simulink model "left_arm_observer"  (R2019b)
settings: Solver=ode4  StartTime=0.0  StopTime=inf  FixedStep=0.001  MaxStep=0.01  RelTol=1e-3
model workspace (MAT data in the model file):
  SL_ROS_VariableLengthArrays_MaxSizes.CommonInfo.ArrayTruncateAction = 'EmitWarning'
  SL_ROS_VariableLengthArrays_MaxSizes.MsgTypeMap = containers.Map
  SL_ROS_VariableLengthArrays_MaxSizes.MsgTypeMap.serialization.keys = {'sensor_msgs/JointState', 'std_msgs/Float64MultiArray', 'std_msgs/String'}
  SL_ROS_VariableLengthArrays_MaxSizes.MsgTypeMap.serialization.values{1}(1).PropertyName = 'Effort'
  SL_ROS_VariableLengthArrays_MaxSizes.MsgTypeMap.serialization.values{1}(1).DataType = 'double'
  SL_ROS_VariableLengthArrays_MaxSizes.MsgTypeMap.serialization.values{1}(1).MaxLength = 7
  SL_ROS_VariableLengthArrays_MaxSizes.MsgTypeMap.serialization.values{1}(2).PropertyName = 'Name'
  SL_ROS_VariableLengthArrays_MaxSizes.MsgTypeMap.serialization.values{1}(2).DataType = 'std_msgs/String'
  SL_ROS_VariableLengthArrays_MaxSizes.MsgTypeMap.serialization.values{1}(2).MaxLength = 7
  SL_ROS_VariableLengthArrays_MaxSizes.MsgTypeMap.serialization.values{1}(3).PropertyName = 'Position'
  SL_ROS_VariableLengthArrays_MaxSizes.MsgTypeMap.serialization.values{1}(3).DataType = 'double'
  SL_ROS_VariableLengthArrays_MaxSizes.MsgTypeMap.serialization.values{1}(3).MaxLength = 7
  SL_ROS_VariableLengthArrays_MaxSizes.MsgTypeMap.serialization.values{1}(4).PropertyName = 'Velocity'
  SL_ROS_VariableLengthArrays_MaxSizes.MsgTypeMap.serialization.values{1}(4).DataType = 'double'
  SL_ROS_VariableLengthArrays_MaxSizes.MsgTypeMap.serialization.values{1}(4).MaxLength = 7
  SL_ROS_VariableLengthArrays_MaxSizes.MsgTypeMap.serialization.values{2}.PropertyName = 'Data'
  SL_ROS_VariableLengthArrays_MaxSizes.MsgTypeMap.serialization.values{2}.DataType = 'double'
  SL_ROS_VariableLengthArrays_MaxSizes.MsgTypeMap.serialization.values{2}.MaxLength = 7
  SL_ROS_VariableLengthArrays_MaxSizes.MsgTypeMap.serialization.values{3}.PropertyName = 'Data'
  SL_ROS_VariableLengthArrays_MaxSizes.MsgTypeMap.serialization.values{3}.DataType = 'uint8'
  SL_ROS_VariableLengthArrays_MaxSizes.MsgTypeMap.serialization.values{3}.MaxLength = 10
  SL_ROS_VariableLengthArrays_MaxSizes.MsgTypeMap.serialization.uniformity = 0
  SL_ROS_VariableLengthArrays_MaxSizes.MsgTypeMap.serialization.keyType = 'char'
  SL_ROS_VariableLengthArrays_MaxSizes.MsgTypeMap.serialization.valueType = 'any'
undefined symbols (not defined in the file or in its folder): Data, Data_SL_Info
libraries: robotlib x5, robotmaniplib x3, robotcorelib x1
settings Model: EnablePacing=on  Creator=marco  LastModifiedBy=marco
settings OptimizationCC: EnhancedBackFolding=on  PassReuseOutputArgsAs=Individual arguments  ZeroExternalMemoryAtStartup=off  ZeroInternalMemoryAtStartup=off  MaxStackSize=64  OptimizeBlockOrder=speed  DifferentSizesBufferReuse=on  OptimizationCustomize=off  EfficientTunableParamExpr=on
settings DebuggingCC: ParameterTunabilityLossMsg=error
settings HardwareCC: ProdBitPerLong=64  ProdHWDeviceType=Intel->x86-64 (Linux 64)
settings RTWCC: SystemTargetFile=ert.tlc  HardwareBoard=Robot Operating System (ROS)  TLCOptions="-aInlineSetEventsForThisBaseRateFcn=TLC_FALSE -aSuppressMultiTaskScheduler=TLC_FALSE  -aRateBasedStepFcn=0"  TemplateMakefile=ert_default_tmf  GenerateReport=on  Toolchain=Catkin  IncludeHyperlinkInReport=on  LaunchReport=on  TargetLang=C++  GenerateTraceInfo=on  GenerateTraceReport=on  GenerateTraceReportSl=on  GenerateTraceReportSf=on  GenerateTraceReportEml=on
settings CodeAppCC: ForceParamTrailComments=on  IgnoreCustomStorageClasses=off  OperatorAnnotations=on  SimulinkDataObjDesc=on  SFDataObjDesc=on  InsertBlockDesc=on
settings ERTTargetCC: SupportContinuousTime=on  SupportVariableSizeSignals=on
settings ExplorerConfigSet: InternalSimMechanicsExplorerSettings="<ExplorerConfiguration><canonicalview>aerospace</canonicalview><AnimationSetting><BasePlaybackSpeed>1.0</BasePlaybackSpeed><PlaybackSpeedFactor>1.0</PlaybackSpeedFactor></AnimationSetting><TilePanel><TileInfo><Tiles Columns=\"1\" Count=\"1\" Rows=\"1\"><Column Weight=\"1\"/><Row Weight=\"1\"/><Tile Height=\"1\" Width=\"1\" X=\"0\" Y=\"0\"/></Tiles></TileInfo><SceneInfo><SceneViewer><BGColor><R>0.60000002384185791</R><G>0.60000002384185791</G><B>0.60000002384185791</B></BGColor><Camera><DoPerspective>off</DoPerspective><Position><X>0.470747241724220999</X><Y>0.672742710715300452</Y><Z>0.803552756362765797</Z></Position><Center><X>0.426167977285198674</X><Y>0.0857009724355916047</Y><Z>-0.00477557216445684274</Z></Center><Up><X>-0.998971998504803671</X><Y>0.0328560329609175472</Y><Z>0.0312318315407420499</Z></Up><ViewLimDist>1</ViewLimDist><YLim>0.446111832261085528</YLim><XLim>0.664557689711664734</XLim></Camera></SceneViewer></SceneInfo></TilePanel><MechEditorPanel><Cameras/><GfxPanelCameraMap/><VideoCreator><PlaybackSpeedRatio>1.0</PlaybackSpeedRatio><FrameRate>30</FrameRate><VideoFormat>Motion JPEG AVI</VideoFormat><FrameSize>auto</FrameSize></VideoCreator></MechEditorPanel></ExplorerConfiguration>"

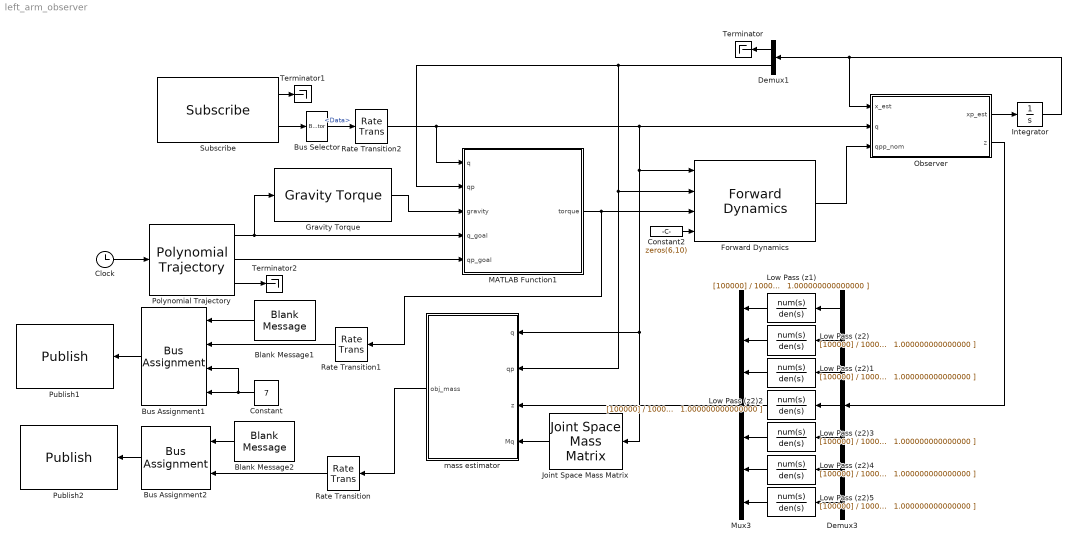
== system left_arm_observer ==
  Blank Message1 : robotlib/Blank Message  messageClass=Message  entityType=std_msgs/Float64MultiArray  messageType=std_msgs/Float64MultiArray  SampleTime=0.001
      settings: SourceProductName=ROS Toolbox
  Blank Message2 : robotlib/Blank Message  messageClass=Message  entityType=std_msgs/Float64  messageType=std_msgs/Float64  SampleTime=0.05
      settings: SourceProductName=ROS Toolbox
  Bus Assignment1 : BusAssignment  AssignedSignals=Data,Data_SL_Info.CurrentLength,Data_SL_Info.ReceivedLength
  Bus Assignment2 : BusAssignment  AssignedSignals=Data
  Bus Selector : BusSelector  OutputSignals=Data
  Clock : Clock
  Constant : Constant  Value=7  OutDataTypeStr=uint32  SampleTime=0.001
  Constant2 : Constant  Value=zeros(6,10)  SampleTime=-1
  Demux1 : Demux  Outputs=[7,7]
  Demux3 : Demux  Outputs=7
  Forward Dynamics : robotmaniplib/Forward Dynamics  RigidBodyTree=justina_left_arm  SimulateUsing=Code generation
      settings: SourceProductName=Robotics System Toolbox
  Gravity Torque : robotmaniplib/Gravity Torque  RigidBodyTree=justina_left_arm  SimulateUsing=Code generation
      settings: SourceProductName=Robotics System Toolbox
  Integrator : Integrator  InitialCondition=[0 0 0 0 0 0 0 0 0 0 0 0 0 0]
  Joint Space Mass Matrix : robotmaniplib/Joint Space Mass Matrix  RigidBodyTree=justina_left_arm  SimulateUsing=Code generation
      settings: SourceProductName=Robotics System Toolbox
  Low Pass (z1) : TransferFcn  Numerator=[100000]  Denominator=|
      | 100000*[0.000010000000000   0.000323606797750   0.005236067977500   0.052360679774998   0.323606797749979   1.000000000000000
      | ]
  Low Pass (z2) : TransferFcn  Numerator=[100000]  Denominator=|
      | 100000*[0.000010000000000   0.000323606797750   0.005236067977500   0.052360679774998   0.323606797749979   1.000000000000000
      | ]
  Low Pass (z2)1 : TransferFcn  Numerator=[100000]  Denominator=|
      | 100000*[0.000010000000000   0.000323606797750   0.005236067977500   0.052360679774998   0.323606797749979   1.000000000000000
      | ]
  Low Pass (z2)2 : TransferFcn  Numerator=[100000]  Denominator=|
      | 100000*[0.000010000000000   0.000323606797750   0.005236067977500   0.052360679774998   0.323606797749979   1.000000000000000
      | ]
  Low Pass (z2)3 : TransferFcn  Numerator=[100000]  Denominator=|
      | 100000*[0.000010000000000   0.000323606797750   0.005236067977500   0.052360679774998   0.323606797749979   1.000000000000000
      | ]
  Low Pass (z2)4 : TransferFcn  Numerator=[100000]  Denominator=|
      | 100000*[0.000010000000000   0.000323606797750   0.005236067977500   0.052360679774998   0.323606797749979   1.000000000000000
      | ]
  Low Pass (z2)5 : TransferFcn  Numerator=[100000]  Denominator=|
      | 100000*[0.000010000000000   0.000323606797750   0.005236067977500   0.052360679774998   0.323606797749979   1.000000000000000
      | ]
  MATLAB Function1 : MATLAB Function  TreatAsAtomicUnit=on
  Mux3 : Mux  Inputs=7
  Observer : MATLAB Function  TreatAsAtomicUnit=on
  Polynomial Trajectory : robotcorelib/Polynomial Trajectory  WaypointSource=Internal  Waypoints=[ 0, -1; 0, 0; 0, 0; 0 1.5; 0, 0; 0, 0.5; 0, 0]  TimePoints=[ 0, 3]  TimeInterval=[ 1, 4 ]  Method=Quintic Polynomial  ParameterSource=Internal  VelocityBoundaryCondition=zeros( 7, 2 )  AccelerationBoundaryCondition=zeros( 7, 2 )  SimulateUsing=Code generation
      settings: SourceProductName=Robotics System Toolbox  SourceProductBaseCode=RO
  Publish1 : robotlib/Publish  topicSource=Specify your own  topic=/hardware/la_torque  messageType=std_msgs/Float64MultiArray  messageQueueLength=1
      settings: SourceProductName=ROS Toolbox
  Publish2 : robotlib/Publish  topicSource=Specify your own  topic=/estimated_mass  messageType=std_msgs/Float64  messageQueueLength=1
      settings: SourceProductName=ROS Toolbox
  Rate Transition : RateTransition
  Rate Transition1 : RateTransition
  Rate Transition2 : RateTransition
  Subscribe : robotlib/Subscribe  topicSource=Specify your own  topic=/hardware/la_current_pose  messageType=std_msgs/Float64MultiArray  sampleTime=0.001  messageQueueLength=1
      settings: SourceProductName=ROS Toolbox
  Terminator : Terminator
  Terminator1 : Terminator
  Terminator2 : Terminator
  mass estimator : MATLAB Function  TreatAsAtomicUnit=on
  wires:
  Demux1/1 -> Terminator/1
  Gravity Torque/1 -> MATLAB Function1/3(gravity)
  Constant2/1 -> Forward Dynamics/4
  Demux3/2 -> Low Pass (z2)/1
  Low Pass (z2)/1 -> Mux3/2
  Low Pass (z1)/1 -> Mux3/1
  Demux3/1 -> Low Pass (z1)/1
  mass estimator/1(obj_mass) -> Rate Transition/1
  Demux1/2 -> MATLAB Function1/2(qp), mass estimator/2(qp), Forward Dynamics/2
  Low Pass (z2)5/1 -> Mux3/7
  Low Pass (z2)4/1 -> Mux3/6
  Low Pass (z2)3/1 -> Mux3/5
  Low Pass (z2)2/1 -> Mux3/4
  Low Pass (z2)1/1 -> Mux3/3
  Demux3/3 -> Low Pass (z2)1/1
  Demux3/4 -> Low Pass (z2)2/1
  Demux3/5 -> Low Pass (z2)3/1
  Demux3/6 -> Low Pass (z2)4/1
  Demux3/7 -> Low Pass (z2)5/1
  Clock/1 -> Polynomial Trajectory/1
  Subscribe/2 -> Bus Selector/1
  Subscribe/1 -> Terminator1/1
  Observer/2(z) -> Demux3/1
  Observer/1(xp_est) -> Integrator/1
  Mux3/1 -> mass estimator/3(z)
  Forward Dynamics/1 -> Observer/3(qpp_nom)
  Polynomial Trajectory/1 -> MATLAB Function1/4(q_goal), Gravity Torque/1
  Integrator/1 -> Demux1/1, Observer/1(x_est)
  Bus Selector/1 -> Rate Transition2/1  "<Data>"
  Joint Space Mass Matrix/1 -> mass estimator/4(Mq)
  Bus Assignment1/1 -> Publish1/1
  Blank Message1/1 -> Bus Assignment1/1
  Constant/1 -> Bus Assignment1/4, Bus Assignment1/3
  MATLAB Function1/1(torque) -> Rate Transition1/1, Forward Dynamics/3
  Polynomial Trajectory/2 -> MATLAB Function1/5(qp_goal)
  Polynomial Trajectory/3 -> Terminator2/1
  Blank Message2/1 -> Bus Assignment2/1
  Rate Transition/1 -> Bus Assignment2/2
  Bus Assignment2/1 -> Publish2/1
  Rate Transition1/1 -> Bus Assignment1/2
  Rate Transition2/1 -> MATLAB Function1/1(q), Joint Space Mass Matrix/1, mass estimator/1(q), Forward Dynamics/1, Observer/2(q)

== matlab function left_arm_observer/mass estimator ==
  data: q input; qp input; z input; obj_mass output; Mq input
function obj_mass = mass_est(q, qp, z, Mq)
phi = Mq*z;
g = 9.81;
l = 0.195;
vel = norm(qp);
%obj_mass = zeros(1,2);
if abs(sin(q(1) + q(4) + q(6))) > 0.1 && vel < 0.1
    obj_mass = -phi(6)/(l*g*sin(q(1) + q(4) + q(6)));
    %obj_mass(2) = -phi(4)/(0.33*9.81*sin(q(1) + q(4)));
else
    obj_mass = 0;
end

== matlab function left_arm_observer/MATLAB Function1 ==
  data: q input; qp input; gravity input; q_goal input; torque output; qp_goal input
function torque = position_control(q,qp, gravity, q_goal, qp_goal)
%%Constantes del control PD
kp=[20.5; 1.0; 1.0; 14.5; 1.0; 10.5; 1.0];
kd=[7.0; 1.0; 1.0; 5.0; 1.0; 5.0; 1.0];

qe = zeros(1,7);
qpe = zeros(1,7);
torque = zeros(1,7);
for i=1:7
    qe(i) = q_goal(i) - q(i);
    qpe(i) = qp_goal(i) - qp(i);
    torque(i) = gravity(i) + kp(i)*qe(i) + kd(i)*qpe(i);
end

== matlab function left_arm_observer/Observer ==
  data: x_est input; q input; qpp_nom input; xp_est output; z output
function [xp_est, z] = observer(x_est, q, qpp_nom)
xp_est = zeros(1,14);
q_est  = x_est(1:7);
qp_est = x_est(8:14);
z1 = zeros(1,7);
z2 = zeros(1,7);

%lambda = 3;
%alpha  = 3;
lambda = 6;
alpha  = 6;

for i=1:7
    z1(i) = lambda*sqrt(abs(q(i) - q_est(i)))*sign(q(i) - q_est(i));
    z2(i) = alpha*sign(q(i) - q_est(i));
end

for i=1:7
    xp_est(i)   = qp_est(i)  + z1(i);
    xp_est(i+7) = qpp_nom(i) + z2(i);
end

z = z2;
